simulink model "rtwdemo_tflscalarops"  (Simulink 7.6)
settings: Solver=FixedStepDiscrete  StartTime=0.0  StopTime=20  FixedStep=.01  RelTol=1e-3  SampleTimeConstraint=Specified
PreLoadFcn:
  | addpath(fullfile(matlabroot,'toolbox','rtw','rtwdemos','tfl_demo'));
  | sl_refresh_customizations;
libraries: simulink x3, rtwdemowidgets x2
settings Model: Creator=The MathWorks Inc.  ExtModeAutoUpdateStatusClock=off
settings MATStruct: SampleTime=1  Offset=0  Priority=[30.0]
settings DataIOCC: SaveOutput=off  SaveTime=off  SignalLoggingName=sigsOut
settings OptimizationCC: InlineParams=on  UseIntDivNetSlope=on  InlineInvariantSignals=on  EnhancedBackFolding=on  BooleansAsBitfields=on  PassReuseOutputArgsAs=Individual arguments  StateBitsets=on  DataBitsets=on  UseTempVars=on  ZeroExternalMemoryAtStartup=off  ZeroInternalMemoryAtStartup=off  NoFixptDivByZeroProtection=on  EfficientFloat2IntCast=on  OptimizeModelRefInitCode=on  LifeSpan=1
settings DebuggingCC: CheckExecutionContextPreStartOutputMsg=on  CheckExecutionContextRuntimeOutputMsg=on  SolverPrmCheckMsg=none  IntegerOverflowMsg=none  StrictBusMsg=ErrorOnBusTreatedAsVector
settings HardwareCC: ProdBitPerLong=64  ProdIntDivRoundTo=Zero  ProdEndianess=LittleEndian  ProdWordSize=64  ProdHWDeviceType=Specified  TargetHWDeviceType=32-bit Generic
settings SFSimCC: SFSimEnableDebug=off  SFSimOverflowDetection=off  SimParseCustomCode=off
settings RTWCC: SystemTargetFile=ert.tlc  TemplateMakefile=ert_default_tmf  Description=Real-Time Workshop Embedded Coder  GenerateReport=on  RTWVerbose=off  ProcessScript=ert_make_rtw_hook  IncludeHyperlinkInReport=on  LaunchReport=on  GenerateTraceInfo=on  GenerateTraceReport=on  GenerateTraceReportSl=on  GenerateTraceReportSf=on  GenerateTraceReportEml=on
settings CodeAppCC: ForceParamTrailComments=on  IgnoreCustomStorageClasses=off  IgnoreTestpoints=on  SimulinkDataObjDesc=on  CustomSymbolStrGlobalVar=rt$N$M  CustomSymbolStrType=$N$M  CustomSymbolStrFcn=$N$M$F  CustomSymbolStrMacro=$N$M  InsertBlockDesc=on
settings ERTTargetCC: TargetFunctionLibrary=Scalar Operation Examples  MultiwordLength=2048  GenerateSampleERTMain=on  IncludeMdlTerminateFcn=off  SupportNonFinite=off  InlinedParameterPlacement=NonHierarchical  ERTCustomFileTemplate=example_file_process.tlc  ConvertIfToSwitch=off

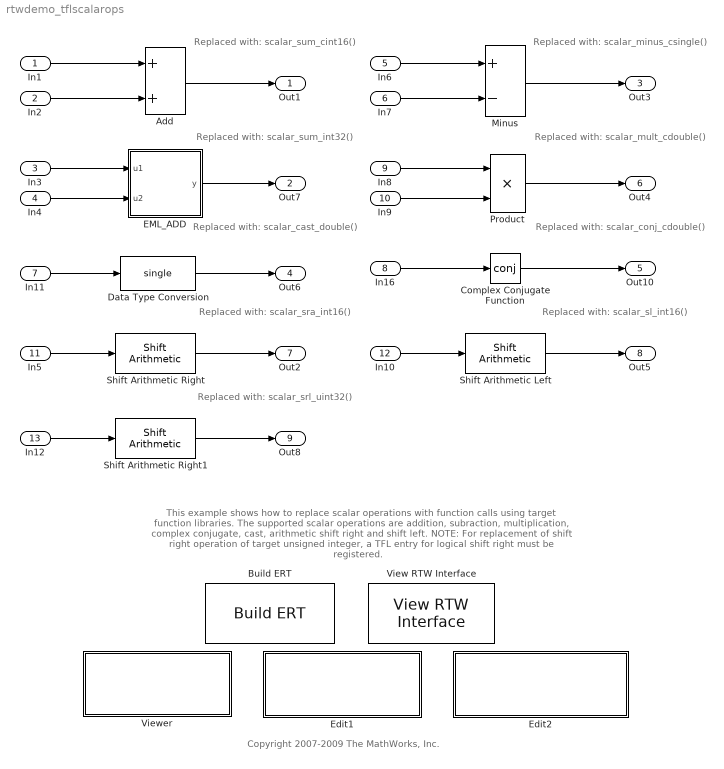
== system rtwdemo_tflscalarops ==
  note: Copyright 2007-2009 The MathWorks, Inc.
  note: Replaced with:
      | scalar_sum_cint16()
  note: Replaced with:
      | scalar_sum_int32()
  note: Replaced with:
      | scalar_minus_csingle()
  note: This example shows how to replace scalar operations with
      | function calls using target function libraries.
      |
      | The supported scalar operations are addition, subraction, multiplication, complex conjugate, cast, arithmetic shift right and shift left.
      | NOTE: For replacement of shift right operation of target unsigned integer, a TFL entry for logical shift right must be registered.
  note: Replaced with:
      | scalar_cast_double()
  note: Replaced with:
      | scalar_conj_cdouble()
  note: Replaced with:
      | scalar_mult_cdouble()
  note: Replaced with:
      | scalar_sra_int16()
  note: Replaced with:
      | scalar_sl_int16()
  note: Replaced with:
      | scalar_srl_uint32()
  In1 : Inport  OutDataTypeStr=int16  SampleTime=1
      settings: SignalType=complex
  In2 : Inport  Port=2  OutDataTypeStr=int16  SampleTime=1
      settings: SignalType=complex
  In3 : Inport  Port=3  OutDataTypeStr=int32  SampleTime=1
  In4 : Inport  Port=4  OutDataTypeStr=int32  SampleTime=1
  In6 : Inport  Port=5  OutDataTypeStr=single  SampleTime=1
      settings: SignalType=complex
  In7 : Inport  Port=6  OutDataTypeStr=single  SampleTime=1
      settings: SignalType=complex
  In11 : Inport  Port=7  OutDataTypeStr=double  SampleTime=1
  In16 : Inport  Port=8  OutDataTypeStr=double  SampleTime=1
      settings: SignalType=complex
  In8 : Inport  Port=9  OutDataTypeStr=double  SampleTime=1
      settings: SignalType=complex
  In9 : Inport  Port=10  OutDataTypeStr=double  SampleTime=1
      settings: SignalType=complex
  In5 : Inport  Port=11  OutDataTypeStr=int16  SampleTime=1
  In10 : Inport  Port=12  OutDataTypeStr=int16  SampleTime=1
  In12 : Inport  Port=13  OutDataTypeStr=uint32  SampleTime=1
  Add : Sum
  Build ERT : rtwdemowidgets/Build ERT  SystemSampleTime=-1  attrib_overrides={'GenFloatMathFcnCalls', 'SupportComplex'}
  Complex Conjugate Function : Math  Operator=conj
  Data Type Conversion : DataTypeConversion  OutDataTypeStr=single
  EML_ADD : Stateflow chart  TreatAsAtomicUnit=on
  Edit1 : Subsystem  mask{attrib_overrides={}}
      mask prompts: attrib_overrides "List of attributes to preserve (cell of strings):"
      mask help: Enter the attributes of the configuration set that you want preserved. Otherwise, the default configuration script will override your current settings.
      settings: OpenFcn=edit('tfl_table_scalarop');
      mask Display:
      | disp(['View/edit TFL Definition\n',...
      | 	  'tfl_table_scalarop.m\n(double-click)'])
  Edit2 : Subsystem  mask{attrib_overrides={}}
      mask prompts: attrib_overrides "List of attributes to preserve (cell of strings):"
      mask help: Enter the attributes of the configuration set that you want preserved. Otherwise, the default configuration script will override your current settings.
      settings: OpenFcn=edit(fullfile(matlabroot,'toolbox','rtw','rtwdemos','tfl_demo', 'sl_customization.m'));
      mask Display:
      | disp(['View/edit TFL Registration\n',...
      | 	  'sl_customization.m\n(double-click)'])
  Minus : Sum  Inputs=+-
  Product : Product  RndMeth=Zero
  Shift Arithmetic Left : simulink/Logic and Bit Operations/Shift Arithmetic  SystemSampleTime=-1  nBitShiftRight=-4  nBinPtShiftRight=0
  Shift Arithmetic Right : simulink/Logic and Bit Operations/Shift Arithmetic  SystemSampleTime=-1  nBitShiftRight=12  nBinPtShiftRight=0
  Shift Arithmetic Right1 : simulink/Logic and Bit Operations/Shift Arithmetic  SystemSampleTime=-1  nBitShiftRight=15  nBinPtShiftRight=0
  View RTW Interface : rtwdemowidgets/View RTW Interface  SystemSampleTime=-1
  Viewer : Subsystem  mask{attrib_overrides={}}
      mask prompts: attrib_overrides "List of attributes to preserve (cell of strings):"
      mask help: Enter the attributes of the configuration set that you want preserved. Otherwise, the default configuration script will override your current settings.
      settings: OpenFcn=|
      | tfl = tfl_table_scalarop;
      | obj = RTW.viewTfl(tfl);
      | clear tfl obj;
      mask Display:
      | disp(['Invoke TFL Viewer on\n',...
      | 	  'tfl_table_scalarop.m\n(double-click)'])
  Out1 : Outport
  Out7 : Outport  Port=2
  Out3 : Outport  Port=3
  Out6 : Outport  Port=4
  Out10 : Outport  Port=5
  Out4 : Outport  Port=6
  Out2 : Outport  Port=7
  Out5 : Outport  Port=8
  Out8 : Outport  Port=9
  wires:
  Add/1 -> Out1/1
  In1/1 -> Add/1
  In2/1 -> Add/2
  EML_ADD/1(y) -> Out7/1
  Minus/1 -> Out3/1
  In4/1 -> EML_ADD/2(u2)
  In6/1 -> Minus/1
  In7/1 -> Minus/2
  Data Type Conversion/1 -> Out6/1
  In11/1 -> Data Type Conversion/1
  Complex Conjugate Function/1 -> Out10/1
  In16/1 -> Complex Conjugate Function/1
  In8/1 -> Product/1
  In9/1 -> Product/2
  Product/1 -> Out4/1
  In5/1 -> Shift Arithmetic Right/1
  Shift Arithmetic Right/1 -> Out2/1
  In10/1 -> Shift Arithmetic Left/1
  Shift Arithmetic Left/1 -> Out5/1
  In3/1 -> EML_ADD/1(u1)
  In12/1 -> Shift Arithmetic Right1/1
  Shift Arithmetic Right1/1 -> Out8/1

== system rtwdemo_tflscalarops/Edit1 ==

== system rtwdemo_tflscalarops/Edit2 ==

== system rtwdemo_tflscalarops/Viewer ==

== matlab function EML_ADD ==
  data: u1 input uint32; y output uint32; u2 input uint32
function y = fcn(u1, u2)
% This block supports the Embedded MATLAB subset.
% See the help menu for details. 

y = u1 + u2;
